simulink model "DSM_MOD8_LTE_HDL"  (R2013b)
settings: Solver=VariableStepAuto  StartTime=0.0  StopTime=1.0  RelTol=1e-3
undefined symbols (not defined in the file or in its folder): a, b, c, g
settings Model: Creator=o_cotte  LastModifiedBy=o_cotte
settings DataIOCC: LimitDataPoints=off  SaveFormat=Dataset
settings OptimizationCC: LifeSpan=auto  SimCompilerOptimization=off
settings DebuggingCC: UnderspecifiedInitializationDetection=Simplified  MergeDetectMultiDrivingBlocksExec=error  SolverPrmCheckMsg=none  FcnCallInpInsideContextMsg=error  FrameProcessingCompatibilityMsg=error  SFUnexpectedBacktrackingDiag=error  SFNoUnconditionalDefaultTransitionDiag=error
settings HardwareCC: ProdBitPerPointer=64  ProdLargestAtomicFloat=Float  ProdIntDivRoundTo=Zero  ProdEndianess=LittleEndian  ProdWordSize=64  ProdHWDeviceType=Intel->x86-64 (Windows64)
settings ModelReferenceCC: PropagateSignalLabelsOutOfModel=on
settings RTWCC: RTWCompilerOptimization=off
settings GRTTargetCC: CodeReplacementLibrary=None  GeneratePreprocessorConditionals=Use local settings  CPPClassGenCompliant=on

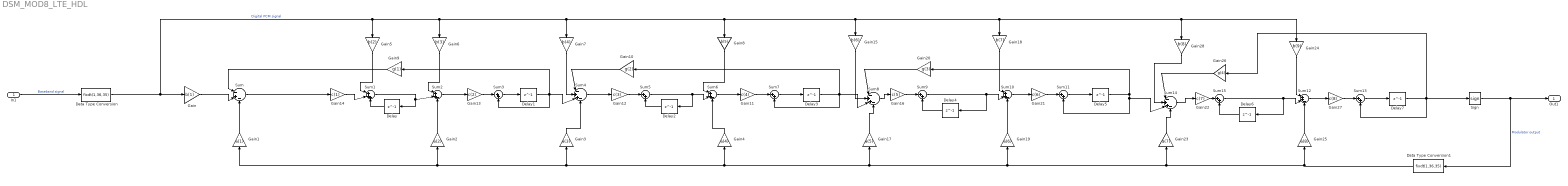
== system DSM_MOD8_LTE_HDL ==
  In1 : Inport
  Data Type Conversion : DataTypeConversion  OutDataTypeStr=fixdt(1,36,35)
  Data Type Conversion1 : DataTypeConversion  OutDataTypeStr=fixdt(1,36,35)
  Delay{,1..7} (8 alike) : Delay  DelayLength=1  InitialCondition=0
  Gain : Gain  Gain=b(1)  OutDataTypeStr=Inherit: Same as input  ParamDataTypeStr=Inherit: Same as input  LockScale=on
  Gain1 : Gain  Gain=a(1)  OutDataTypeStr=Inherit: Same as input
  Gain10 : Gain  Gain=g(2)  OutDataTypeStr=Inherit: Same as input  ParamDataTypeStr=Inherit: Same as input  LockScale=on
  Gain11 : Gain  Gain=c(4)  OutDataTypeStr=Inherit: Same as input  ParamDataTypeStr=Inherit: Same as input  LockScale=on
  Gain12 : Gain  Gain=c(3)  OutDataTypeStr=Inherit: Same as input  ParamDataTypeStr=Inherit: Same as input  LockScale=on
  Gain13 : Gain  Gain=c(2)  OutDataTypeStr=Inherit: Same as input  ParamDataTypeStr=Inherit: Same as input  LockScale=on
  Gain14 : Gain  Gain=c(1)  OutDataTypeStr=Inherit: Same as input  ParamDataTypeStr=Inherit: Same as input  LockScale=on
  Gain15 : Gain  Gain=b(6)  OutDataTypeStr=Inherit: Same as input  ParamDataTypeStr=Inherit: Same as input  LockScale=on
  Gain16 : Gain  Gain=c(5)  OutDataTypeStr=Inherit: Same as input  ParamDataTypeStr=Inherit: Same as input  LockScale=on
  Gain17 : Gain  Gain=a(5)  OutDataTypeStr=Inherit: Same as input
  Gain18 : Gain  Gain=b(7)  OutDataTypeStr=Inherit: Same as input  ParamDataTypeStr=Inherit: Same as input  LockScale=on
  Gain19 : Gain  Gain=a(6)  OutDataTypeStr=Inherit: Same as input
  Gain2 : Gain  Gain=a(2)  OutDataTypeStr=Inherit: Same as input
  Gain20 : Gain  Gain=g(3)  OutDataTypeStr=Inherit: Same as input  ParamDataTypeStr=Inherit: Same as input  LockScale=on
  Gain21 : Gain  Gain=c(6)  OutDataTypeStr=Inherit: Same as input  ParamDataTypeStr=Inherit: Same as input  LockScale=on
  Gain22 : Gain  Gain=c(7)  OutDataTypeStr=Inherit: Same as input  ParamDataTypeStr=Inherit: Same as input  LockScale=on
  Gain23 : Gain  Gain=a(7)  OutDataTypeStr=Inherit: Same as input
  Gain24 : Gain  Gain=b(9)  OutDataTypeStr=Inherit: Same as input  ParamDataTypeStr=Inherit: Same as input  LockScale=on
  Gain25 : Gain  Gain=a(8)  OutDataTypeStr=Inherit: Same as input
  Gain26 : Gain  Gain=g(4)  OutDataTypeStr=Inherit: Same as input  ParamDataTypeStr=Inherit: Same as input  LockScale=on
  Gain27 : Gain  Gain=c(8)  OutDataTypeStr=Inherit: Same as input  ParamDataTypeStr=Inherit: Same as input  LockScale=on
  Gain28 : Gain  Gain=b(8)  OutDataTypeStr=Inherit: Same as input  ParamDataTypeStr=Inherit: Same as input  LockScale=on
  Gain3 : Gain  Gain=a(3)  OutDataTypeStr=Inherit: Same as input
  Gain4 : Gain  Gain=a(4)  OutDataTypeStr=Inherit: Same as input
  Gain5 : Gain  Gain=b(2)  OutDataTypeStr=Inherit: Same as input  ParamDataTypeStr=Inherit: Same as input  LockScale=on
  Gain6 : Gain  Gain=b(3)  OutDataTypeStr=Inherit: Same as input  ParamDataTypeStr=Inherit: Same as input  LockScale=on
  Gain7 : Gain  Gain=b(4)  OutDataTypeStr=Inherit: Same as input  ParamDataTypeStr=Inherit: Same as input  LockScale=on
  Gain8 : Gain  Gain=b(5)  OutDataTypeStr=Inherit: Same as input  ParamDataTypeStr=Inherit: Same as input  LockScale=on
  Gain9 : Gain  Gain=g(1)  OutDataTypeStr=Inherit: Same as input  ParamDataTypeStr=Inherit: Same as input  LockScale=on
  Sign : Signum
  Sum : Sum  Inputs=|-+-  OutDataTypeStr=Inherit: Same as accumulator  LockScale=on
  Sum1 : Sum  Inputs=|+++  OutDataTypeStr=Inherit: Same as accumulator  LockScale=on
  Sum{2,6,10,12} (4 alike) : Sum  Inputs=|++-  OutDataTypeStr=Inherit: Same as accumulator  LockScale=on
  Sum{3,5,7,9,11,13,15} (7 alike) : Sum  Inputs=|++  OutDataTypeStr=Inherit: Same as accumulator  LockScale=on
  Sum14 : Sum  Inputs=|-++-  OutDataTypeStr=Inherit: Same as accumulator  LockScale=on
  Sum4 : Sum  Inputs=|-++-  OutDataTypeStr=Inherit: Same as accumulator  LockScale=on
  Sum8 : Sum  Inputs=|-++-  OutDataTypeStr=Inherit: Same as accumulator  LockScale=on
  Out1 : Outport
  wires:
  Sum/1 -> Gain14/1
  Gain/1 -> Sum/2
  In1/1 -> Data Type Conversion/1  "Baseband signal"
  Gain1/1 -> Sum/3
  Gain2/1 -> Sum2/3
  Gain3/1 -> Sum4/4
  Gain4/1 -> Sum6/3
  Sum3/1 -> Delay1/1
  Sum7/1 -> Delay3/1
  Sum1/1 -> Delay/1, Sum2/2
  Delay1/1 -> Sum3/2, Gain9/1, Sum4/3
  Sum5/1 -> Delay2/1, Sum6/2
  Gain5/1 -> Sum1/1
  Sum2/1 -> Gain13/1
  Gain6/1 -> Sum2/1
  Gain7/1 -> Sum4/2
  Gain8/1 -> Sum6/1
  Sum6/1 -> Gain11/1
  Sum4/1 -> Gain12/1
  Delay/1 -> Sum1/3
  Delay2/1 -> Sum5/2
  Gain10/1 -> Sum4/1
  Delay3/1 -> Sum8/3, Sum7/2, Gain10/1
  Gain9/1 -> Sum/1
  Gain11/1 -> Sum7/1
  Gain12/1 -> Sum5/1
  Gain13/1 -> Sum3/1
  Gain14/1 -> Sum1/2
  Gain15/1 -> Sum8/2
  Sum8/1 -> Gain16/1
  Gain17/1 -> Sum8/4
  Gain16/1 -> Sum9/1
  Delay4/1 -> Sum9/2
  Sum9/1 -> Delay4/1, Sum10/2
  Gain18/1 -> Sum10/1
  Gain19/1 -> Sum10/3
  Sum10/1 -> Gain21/1
  Sum11/1 -> Delay5/1
  Gain20/1 -> Sum8/1
  Gain21/1 -> Sum11/1
  Sum14/1 -> Gain22/1
  Gain23/1 -> Sum14/4
  Gain27/1 -> Sum13/1
  Gain26/1 -> Sum14/1
  Sum13/1 -> Delay7/1
  Sign/1 -> Data Type Conversion1/1, Out1/1  "Modulator output"
  Sum12/1 -> Gain27/1
  Sum15/1 -> Delay6/1, Sum12/2
  Data Type Conversion/1 -> Gain5/1, Gain8/1, Gain18/1, Gain28/1, Gain24/1, Gain15/1, Gain7/1, Gain6/1, Gain/1  "Digital PCM signal"
  Gain25/1 -> Sum12/3
  Delay6/1 -> Sum15/2
  Delay5/1 -> Sum14/3, Sum11/2, Gain20/1
  Gain22/1 -> Sum15/1
  Delay7/1 -> Sign/1, Sum13/2, Gain26/1
  Gain24/1 -> Sum12/1
  Gain28/1 -> Sum14/2
  Data Type Conversion1/1 -> Gain25/1, Gain1/1, Gain2/1, Gain3/1, Gain4/1, Gain17/1, Gain19/1, Gain23/1
